simulink model "do_an_tn_ks"  (R2023b)
settings: Solver=VariableStepDiscrete  StartTime=0.0  StopTime=2  MaxStep=1e-7  RelTol=1e-3
values from neighbouring files (symbols this model uses):
  anpha = Vmax^3/(2*Ve*Vmax^2-2*Ve^3)    [daks_delay.m]
  b1 = 2-(wh*Ts1)^2    (= 1.99975325989)    [daks_delay.m]
  b2 = -1    [daks_delay.m]
  b3 = kprv1    [daks_delay.m]
  b4 = kirv1*Ts1+kprv1*((wh*Ts1)^2-2)    [daks_delay.m]
  b5 = kprv1-kirv1*Ts1    [daks_delay.m]
  C = Cmin    [daks_delay.m]
  c1 = 1    [daks_delay.m]
  c2 = kpi+kii*Ts/2    [daks_delay.m]
  c3 = kii*Ts/2-kpi    [daks_delay.m]
  Cf = 20e-6    (= 2e-05)    [daks_delay.m]
  ki1 = Ve/(sqrt(2)*Pe1)    [daks_delay.m]
  ki2 = Ve/(sqrt(2)*Pe2)    [daks_delay.m]
  kv = Vmax/sqrt(2)    [daks_delay.m]
  L = 1.3e-3    (= 0.0013)    [daks_delay.m]
  m4 = (4*m1/Ts^2+2*m2/Ts+m3)/(4*n1/Ts^2+2*n2/Ts+n3)    [daks_delay.m]
  m5 = (-8*m1/Ts^2+2*m3)/(4*n1/Ts^2+2*n2/Ts+n3)    [daks_delay.m]
  m6 = (4*m1/Ts^2-2*m2/Ts+m3)/(4*n1/Ts^2+2*n2/Ts+n3)    [daks_delay.m]
  n5 = -(-8*n1/Ts^2+2*n3)/(4*n1/Ts^2+2*n2/Ts+n3)    [daks_delay.m]
  n6 = -(4*n1/Ts^2-2*n2/Ts+n3)/(4*n1/Ts^2+2*n2/Ts+n3)    [daks_delay.m]
  o = 2*anpha    [daks_delay.m]
  Rf = 0.3    [daks_delay.m]
  sw = 4    [daks_delay.m]
  sw1 = 20    [daks_delay.m]
  Ts = 1/20000    (= 5e-05)    [daks_delay.m]
  Udc = 100    [daks_delay.m]
  wnom = 2*pi*50    (= 314.159265359)    [daks_delay.m]
undefined symbols (not defined in the file or in its folder): den_nz1, den_nz2, DiscIntNeverNeededParam, do_an_tn_ks, Down, i, m, num_nz1, num_nz2, Up
libraries: prociolib x12, peripheralslib x12, spsCurrentMeasurementLib x8, spsIGBTDiodeLib x8, spsSeriesRLCBranchLib x7, simulink x6, spsVoltageMeasurementLib x5, spsBreakerLib x2, simulink_extras x2, spsPowerLib x2, spsDCVoltageSourceLib x2, spsSeriesRLCLoadLib x1
(part 2 of 2)

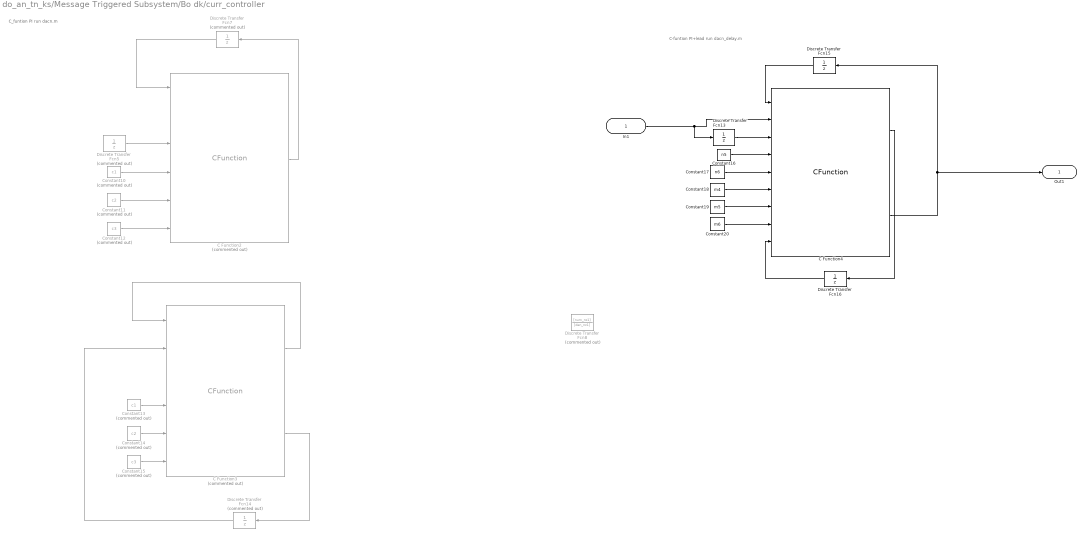
== system do_an_tn_ks/Message Triggered Subsystem/Bo dk/curr_controller ==
  note: C_funtion PI
      |  run dacn.m
  note: C-funtion PI+lead
      | run dacn_delay.m
  In1 : Inport  OutDataTypeStr=double
  C Function2 : CFunction  Commented=on  OutputCode=y_k=c1*y_k_1+c2*u_k+c3*u_k_1;
  C Function3 : CFunction  Commented=on  OutputCode=|  SampleTime=Ts
      | u_k=c2*e_k+v_k_1;
      | v_k=c3*e_k+c1*u_k;
  C Function4 : CFunction  OutputCode=|
      | y_k=m4*u_k+v_k_1;
      | v_k=n5*y_k+n6*y_k_1+m5*u_k+m6*u_k_1;
  Constant10 : Constant  Commented=on  Value=c1  OutDataTypeStr=double
  Constant11 : Constant  Commented=on  Value=c2  OutDataTypeStr=double  SampleTime=-1
  Constant12 : Constant  Commented=on  Value=c3  OutDataTypeStr=double  SampleTime=-1
  Constant13 : Constant  Commented=on  Value=c1  OutDataTypeStr=double
  Constant14 : Constant  Commented=on  Value=c2  OutDataTypeStr=double  SampleTime=-1
  Constant15 : Constant  Commented=on  Value=c3  OutDataTypeStr=double  SampleTime=-1
  Constant16 : Constant  Value=n5  OutDataTypeStr=double
  Constant17 : Constant  Value=n6  OutDataTypeStr=double  SampleTime=-1
  Constant18 : Constant  Value=m4  OutDataTypeStr=double  SampleTime=-1
  Constant19 : Constant  Value=m5  OutDataTypeStr=double  SampleTime=-1
  Constant20 : Constant  Value=m6  OutDataTypeStr=double  SampleTime=-1
  Discrete Transfer Fcn13 : DiscreteTransferFcn  Denominator=[1 0]
  Discrete Transfer Fcn14 : DiscreteTransferFcn  Commented=on  Denominator=[1 0]  SampleTime=Ts
  Discrete Transfer Fcn15 : DiscreteTransferFcn  Denominator=[1 0]
  Discrete Transfer Fcn16 : DiscreteTransferFcn  Denominator=[1 0]
  Discrete Transfer Fcn5 : DiscreteTransferFcn  Commented=on  Denominator=[1 0]
  Discrete Transfer Fcn7 : DiscreteTransferFcn  Commented=on  Denominator=[1 0]
  Discrete Transfer Fcn8 : DiscreteTransferFcn  Commented=on  Numerator=[num_nz1]  Denominator=[den_nz1]  SampleTime=Ts
  Out1 : Outport  OutDataTypeStr=double
  wires:
  C Function2/1 -> Discrete Transfer Fcn7/1
  Constant10/1 -> C Function2/4
  Constant11/1 -> C Function2/5
  Constant12/1 -> C Function2/6
  Discrete Transfer Fcn5/1 -> C Function2/3
  Discrete Transfer Fcn7/1 -> C Function2/1
  C Function3/1 -> C Function3/1
  Constant15/1 -> C Function3/6
  Constant14/1 -> C Function3/5
  Constant13/1 -> C Function3/4
  C Function3/2 -> Discrete Transfer Fcn14/1
  Discrete Transfer Fcn14/1 -> C Function3/2
  Discrete Transfer Fcn16/1 -> C Function4/9
  Discrete Transfer Fcn13/1 -> C Function4/3
  Discrete Transfer Fcn15/1 -> C Function4/1
  Constant16/1 -> C Function4/4
  Constant17/1 -> C Function4/5
  Constant18/1 -> C Function4/6
  Constant19/1 -> C Function4/7
  Constant20/1 -> C Function4/8
  C Function4/2 -> Discrete Transfer Fcn15/1, Out1/1
  C Function4/1 -> Discrete Transfer Fcn16/1
  In1/1 -> Discrete Transfer Fcn13/1, C Function4/2

== system do_an_tn_ks/Message Triggered Subsystem/Bo dk/voltage_controller ==
  In1 : Inport
  C Function1 : CFunction  OutputCode=|
      | y_k=b3*u_k+v_k_1;
      | v_k=b1*y_k+b2*y_k_1+b4*u_k+b5*u_k_1;
  Constant5 : Constant  Value=b1
  Constant6 : Constant  Value=b2
  Constant7 : Constant  Value=b3
  Constant8 : Constant  Value=b4
  Constant9 : Constant  Value=b5
  Discrete Transfer Fcn2 : DiscreteTransferFcn  Denominator=[1 0]
  Discrete Transfer Fcn3 : DiscreteTransferFcn  Denominator=[1 0]
  Discrete Transfer Fcn5 : DiscreteTransferFcn  Denominator=[1 0]
  Discrete Transfer Fcn8 : DiscreteTransferFcn  Commented=on  Numerator=[num_nz2]  Denominator=[den_nz2]  SampleTime=Ts
  Out1 : Outport
  wires:
  Discrete Transfer Fcn2/1 -> C Function1/1
  C Function1/1 -> Discrete Transfer Fcn2/1, Out1/1
  Discrete Transfer Fcn5/1 -> C Function1/3
  Constant5/1 -> C Function1/4
  Constant6/1 -> C Function1/5
  Constant7/1 -> C Function1/6
  Constant8/1 -> C Function1/7
  Constant9/1 -> C Function1/8
  C Function1/2 -> Discrete Transfer Fcn3/1
  Discrete Transfer Fcn3/1 -> C Function1/9
  In1/1 -> C Function1/2, Discrete Transfer Fcn5/1

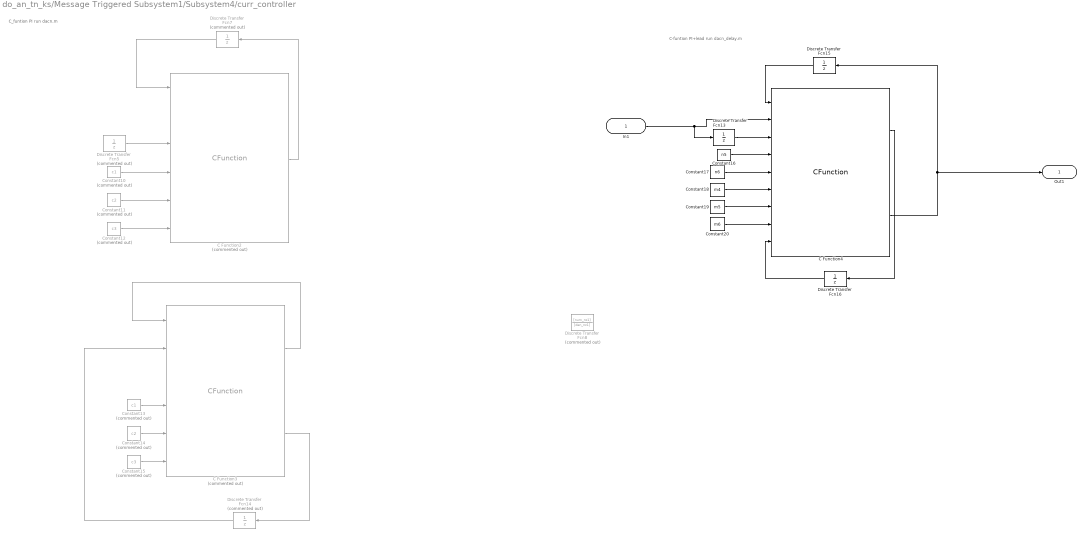
== system do_an_tn_ks/Message Triggered Subsystem1/Subsystem4/curr_controller ==
  note: C-funtion PI+lead
      | run dacn_delay.m
  note: C_funtion PI
      |  run dacn.m
  In1 : Inport  OutDataTypeStr=double
  C Function2 : CFunction  Commented=on  OutputCode=y_k=c1*y_k_1+c2*u_k+c3*u_k_1;
  C Function3 : CFunction  Commented=on  OutputCode=|  SampleTime=Ts
      | u_k=c2*e_k+v_k_1;
      | v_k=c3*e_k+c1*u_k;
  C Function4 : CFunction  OutputCode=|
      | y_k=m4*u_k+v_k_1;
      | v_k=n5*y_k+n6*y_k_1+m5*u_k+m6*u_k_1;
  Constant10 : Constant  Commented=on  Value=c1  OutDataTypeStr=double
  Constant11 : Constant  Commented=on  Value=c2  OutDataTypeStr=double  SampleTime=-1
  Constant12 : Constant  Commented=on  Value=c3  OutDataTypeStr=double  SampleTime=-1
  Constant13 : Constant  Commented=on  Value=c1  OutDataTypeStr=double
  Constant14 : Constant  Commented=on  Value=c2  OutDataTypeStr=double  SampleTime=-1
  Constant15 : Constant  Commented=on  Value=c3  OutDataTypeStr=double  SampleTime=-1
  Constant16 : Constant  Value=n5  OutDataTypeStr=double
  Constant17 : Constant  Value=n6  OutDataTypeStr=double  SampleTime=-1
  Constant18 : Constant  Value=m4  OutDataTypeStr=double  SampleTime=-1
  Constant19 : Constant  Value=m5  OutDataTypeStr=double  SampleTime=-1
  Constant20 : Constant  Value=m6  OutDataTypeStr=double  SampleTime=-1
  Discrete Transfer Fcn13 : DiscreteTransferFcn  Denominator=[1 0]
  Discrete Transfer Fcn14 : DiscreteTransferFcn  Commented=on  Denominator=[1 0]  SampleTime=Ts
  Discrete Transfer Fcn15 : DiscreteTransferFcn  Denominator=[1 0]
  Discrete Transfer Fcn16 : DiscreteTransferFcn  Denominator=[1 0]
  Discrete Transfer Fcn5 : DiscreteTransferFcn  Commented=on  Denominator=[1 0]
  Discrete Transfer Fcn7 : DiscreteTransferFcn  Commented=on  Denominator=[1 0]
  Discrete Transfer Fcn8 : DiscreteTransferFcn  Commented=on  Numerator=[num_nz1]  Denominator=[den_nz1]  SampleTime=Ts
  Out1 : Outport  OutDataTypeStr=double
  wires:
  In1/1 -> C Function4/2, Discrete Transfer Fcn13/1
  C Function4/1 -> Discrete Transfer Fcn16/1
  C Function4/2 -> Out1/1, Discrete Transfer Fcn15/1
  Constant20/1 -> C Function4/8
  Constant19/1 -> C Function4/7
  Constant18/1 -> C Function4/6
  Constant17/1 -> C Function4/5
  Constant16/1 -> C Function4/4
  Discrete Transfer Fcn15/1 -> C Function4/1
  Discrete Transfer Fcn13/1 -> C Function4/3
  Discrete Transfer Fcn16/1 -> C Function4/9
  Discrete Transfer Fcn14/1 -> C Function3/2
  C Function3/2 -> Discrete Transfer Fcn14/1
  Constant13/1 -> C Function3/4
  Constant14/1 -> C Function3/5
  Constant15/1 -> C Function3/6
  C Function3/1 -> C Function3/1
  Discrete Transfer Fcn7/1 -> C Function2/1
  Discrete Transfer Fcn5/1 -> C Function2/3
  Constant12/1 -> C Function2/6
  Constant11/1 -> C Function2/5
  Constant10/1 -> C Function2/4
  C Function2/1 -> Discrete Transfer Fcn7/1

== system do_an_tn_ks/Message Triggered Subsystem1/Subsystem4/voltage_controller ==
  In1 : Inport
  C Function1 : CFunction  OutputCode=|
      | y_k=b3*u_k+v_k_1;
      | v_k=b1*y_k+b2*y_k_1+b4*u_k+b5*u_k_1;
  Constant5 : Constant  Value=b1
  Constant6 : Constant  Value=b2
  Constant7 : Constant  Value=b3
  Constant8 : Constant  Value=b4
  Constant9 : Constant  Value=b5
  Discrete Transfer Fcn2 : DiscreteTransferFcn  Denominator=[1 0]
  Discrete Transfer Fcn3 : DiscreteTransferFcn  Denominator=[1 0]
  Discrete Transfer Fcn5 : DiscreteTransferFcn  Denominator=[1 0]
  Discrete Transfer Fcn8 : DiscreteTransferFcn  Commented=on  Numerator=[num_nz2]  Denominator=[den_nz2]  SampleTime=Ts
  Out1 : Outport
  wires:
  In1/1 -> Discrete Transfer Fcn5/1, C Function1/2
  Discrete Transfer Fcn3/1 -> C Function1/9
  C Function1/2 -> Discrete Transfer Fcn3/1
  Constant9/1 -> C Function1/8
  Constant8/1 -> C Function1/7
  Constant7/1 -> C Function1/6
  Constant6/1 -> C Function1/5
  Constant5/1 -> C Function1/4
  Discrete Transfer Fcn5/1 -> C Function1/3
  C Function1/1 -> Out1/1, Discrete Transfer Fcn2/1
  Discrete Transfer Fcn2/1 -> C Function1/1

== matlab function do_an_tn_ks/Message Triggered Subsystem1/VOC 3/MATLAB Function ==
  data: u input; y output; anpha input; wnom input; i input; kv input; ki input; C input; o input
function y = hopf(u ,anpha ,wnom,i,kv,ki,C,o )
%hopf nolinear oscilator
x1 = u(1); %va
x2 = u(2); %vb

dva = (kv^2*o/anpha-x1^2-x2^2)*x1*anpha/(C*kv^2)-wnom*x2-ki*kv*i/C;
dvb = wnom*x1;
y = [dva;dvb];

== stateflow chart do_an_tn_ks/Message Triggered Subsystem1/Subsystem/Chart1 ==
  state Off
    En_Relay = false;
    enable_bdk = false;
    if (Vout_Rms < 10)
    Grid_Off = Grid_Off + 1;
    Grid_On = 0;
    else
    Grid_On = Grid_On + 1;
    Grid_Off = 0;
    end
  state On_Normal
    En_Relay = true;
    enable_bdk = true;
  state Pre_Synchronous
    En_Relay = false;
    enable_bdk = true;
    if (Error_RMS < 5)
    Change_status = Change_status+1;
    else
    Change_status = 0;
    end
  (default) -> Off
  Off -> On_Normal [order 1] : [Inverter_OnOff == true && Grid_Off >1000]
  On_Normal -> Off : [Inverter_OnOff == false]
  Off -> Pre_Synchronous [order 2] : [Inverter_OnOff == true && Grid_On >1000]
  Pre_Synchronous -> Off [order 2] : [Inverter_OnOff == false]
  Pre_Synchronous -> On_Normal [order 1] : [Change_status > 1000 && Vc1_abs < 10]
  data: Error_RMS input; Inverter_OnOff input; Vout_Rms input; Vc1_abs input; En_Relay output =false; Change_status local =0; Grid_Off local =0; Grid_On local =0; enable_bdk output boolean

== matlab function do_an_tn_ks/Message Triggered Subsystem/VOC 3/MATLAB Function ==
  data: u input; y output; anpha input; wnom input; i input; kv input; ki input; C input; o input
function y = hopf(u ,anpha ,wnom,i,kv,ki,C,o )
%hopf nolinear oscilator
x1 = u(1); %va
x2 = u(2); %vb

dva = (kv^2*o/anpha-x1^2-x2^2)*x1*anpha/(C*kv^2)-wnom*x2-ki*kv*i/C;
dvb = wnom*x1;
y = [dva;dvb];

== matlab function do_an_tn_ks/Message Triggered Subsystem/Subsystem/MATLAB Function ==
  data: vin input; Vrms output; theta output
function [Vrms, theta] = single_phase_rms_phase(vin)
%#codegen

persistent v_alpha v_beta
persistent k w Ts

if isempty(v_alpha)
    v_alpha = 0;
    v_beta  = 0;
    
    Ts = 0.5e-4;          % sampling time (10 kHz -> sửa theo bạn)
    w  = 2*pi*50;       % tần số danh định 50Hz
    k  = sqrt(2);       % gain SOGI
end

% ---- SOGI ----
e = vin - v_alpha;

v_alpha = v_alpha + Ts*( k*w*e - w*v_beta );
v_beta  = v_beta  + Ts*( w*v_alpha );

% ---- RMS ----
Vrms = sqrt( (v_alpha*v_alpha + v_beta*v_beta)/2 );

% ---- Phase ----
theta = atan2(v_beta , v_alpha);

end

== matlab function do_an_tn_ks/Message Triggered Subsystem1/Subsystem/MATLAB Function ==
  data: vin input; Vrms output; theta output
function [Vrms, theta] = single_phase_rms_phase(vin)
%#codegen

persistent v_alpha v_beta
persistent k w Ts

if isempty(v_alpha)
    v_alpha = 0;
    v_beta  = 0;
    
    Ts = 0.5e-4;          % sampling time (10 kHz -> sửa theo bạn)
    w  = 2*pi*50;       % tần số danh định 50Hz
    k  = sqrt(2);       % gain SOGI
end

% ---- SOGI ----
e = vin - v_alpha;

v_alpha = v_alpha + Ts*( k*w*e - w*v_beta );
v_beta  = v_beta  + Ts*( w*v_alpha );

% ---- RMS ----
Vrms = sqrt( (v_alpha*v_alpha + v_beta*v_beta)/2 );

% ---- Phase ----
theta = atan2(v_beta , v_alpha);

end

== matlab function do_an_tn_ks/Message Triggered Subsystem/Subsystem/MATLAB Function1 ==
  data: vin input; Vrms output; theta output
function [Vrms, theta] = single_phase_rms_phase(vin)
%#codegen

persistent v_alpha v_beta
persistent k w Ts

if isempty(v_alpha)
    v_alpha = 0;
    v_beta  = 0;
    
    Ts = 0.5e-4;          % sampling time (10 kHz -> sửa theo bạn)
    w  = 2*pi*50;       % tần số danh định 50Hz
    k  = sqrt(2);       % gain SOGI
end

% ---- SOGI ----
e = vin - v_alpha;

v_alpha = v_alpha + Ts*( k*w*e - w*v_beta );
v_beta  = v_beta  + Ts*( w*v_alpha );

% ---- RMS ----
Vrms = sqrt( (v_alpha*v_alpha + v_beta*v_beta)/2 );

% ---- Phase ----
theta = atan2(v_beta , v_alpha);

end

== matlab function do_an_tn_ks/Message Triggered Subsystem1/Subsystem/MATLAB Function1 ==
  data: vin input; Vrms output; theta output
function [Vrms, theta] = single_phase_rms_phase(vin)
%#codegen

persistent v_alpha v_beta
persistent k w Ts

if isempty(v_alpha)
    v_alpha = 0;
    v_beta  = 0;
    
    Ts = 0.5e-4;          % sampling time (10 kHz -> sửa theo bạn)
    w  = 2*pi*50;       % tần số danh định 50Hz
    k  = sqrt(2);       % gain SOGI
end

% ---- SOGI ----
e = vin - v_alpha;

v_alpha = v_alpha + Ts*( k*w*e - w*v_beta );
v_beta  = v_beta  + Ts*( w*v_alpha );

% ---- RMS ----
Vrms = sqrt( (v_alpha*v_alpha + v_beta*v_beta)/2 );

% ---- Phase ----
theta = atan2(v_beta , v_alpha);

end

== stateflow chart do_an_tn_ks/Message Triggered Subsystem/Subsystem/Chart1 ==
  state Off
    En_Relay = false;
    enable_bdk = false;
    if (Vout_Rms < 10)
    Grid_Off = Grid_Off + 1;
    Grid_On = 0;
    else
    Grid_On = Grid_On + 1;
    Grid_Off = 0;
    end
  state On_Normal
    En_Relay = true;
    enable_bdk = true;
  state Pre_Synchronous
    En_Relay = false;
    enable_bdk = true;
    if (Error_RMS < 5)
    Change_status = Change_status+1;
    else
    Change_status = 0;
    end
  (default) -> Off
  Off -> On_Normal [order 1] : [Inverter_OnOff == true && Grid_Off >1000]
  On_Normal -> Off : [Inverter_OnOff == false]
  Off -> Pre_Synchronous [order 2] : [Inverter_OnOff == true && Grid_On >1000]
  Pre_Synchronous -> Off [order 2] : [Inverter_OnOff == false]
  Pre_Synchronous -> On_Normal [order 1] : [Change_status > 1000 && Vc1_abs < 10]
  data: Error_RMS input; Inverter_OnOff input; Vout_Rms input; Vc1_abs input; En_Relay output =false; Change_status local =0; Grid_Off local =0; Grid_On local =0; enable_bdk output boolean
